simulink model "FruitSorting_slice_fsm"  (R2025a)
settings: Solver=FixedStepDiscrete  StartTime=0.0  StopTime=30  FixedStep=0.05  RelTol=1e-3
undefined symbols (not defined in the file or in its folder): DiscIntNeverNeededParam
settings Model: Creator=Mugin  LastModifiedBy=Mugin

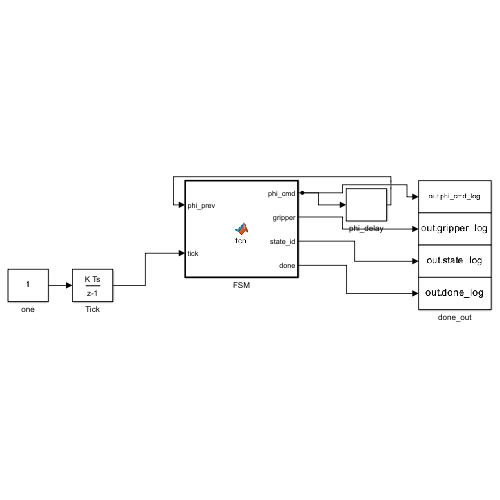
[thumbnail: Simulink's stored preview of the top-level diagram]
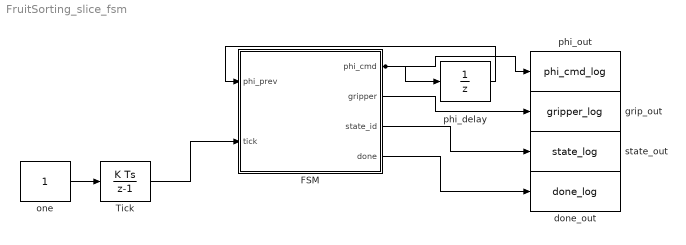
== system FruitSorting_slice_fsm ==
  FSM : MATLAB Function  TreatAsAtomicUnit=on
  Tick : DiscreteIntegrator  gainval=1  SampleTime=0.05  ICPrevOutput=DiscIntNeverNeededParam  ICPrevScaledInput=DiscIntNeverNeededParam
  done_out : ToWorkspace  VariableName=done_log  SampleTime=-1
  grip_out : ToWorkspace  VariableName=gripper_log  SampleTime=-1
  one : Constant  SampleTime=0.05
  phi_delay : UnitDelay  InitialCondition=[0;0;0;0]  SampleTime=0.05  HasFrameUpgradeWarning=on
  phi_out : ToWorkspace  VariableName=phi_cmd_log  SampleTime=-1
  state_out : ToWorkspace  VariableName=state_log  SampleTime=-1
  wires:
  one/1 -> Tick/1
  Tick/1 -> FSM/2(tick)
  phi_delay/1 -> FSM/1(phi_prev)
  FSM/1(phi_cmd) -> phi_delay/1, phi_out/1
  FSM/2(gripper) -> grip_out/1
  FSM/3(state_id) -> state_out/1
  FSM/4(done) -> done_out/1

== matlab function FruitSorting_slice_fsm/FSM ==
  data: phi_prev input; phi_cmd output; tick input; gripper output; state_id output; done output
function [phi_cmd, gripper, state_id, done] = fcn(phi_prev, tick)
%#codegen
coder.extrinsic('py_controller');
phi_cmd = zeros(4,1);
gripper = 0;
state_id = int32(0);
done = int32(0);
reset_flag = double(tick == 0);
[phi_tmp, g_tmp, s_tmp, d_tmp] = py_controller(phi_prev, 0.0500, reset_flag);
phi_cmd = double(phi_tmp);
gripper = double(g_tmp);
state_id = int32(s_tmp);
done = int32(d_tmp);
end
